simulink model "ClassDemo"  (R2014b)
settings: Solver=ode45  StartTime=0.0  StopTime=140  MaxStep=0.1  RelTol=1e-3
libraries: simulink x1
settings Model: Creator=jeff  LastModifiedBy=jeff

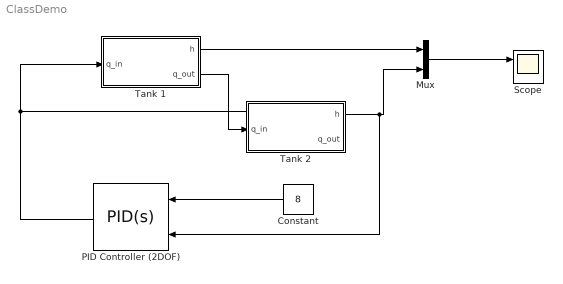
== system ClassDemo ==
  Constant : Constant  Value=8
  Mux : Mux  Inputs=2
  PID Controller (2DOF) : simulink/Continuous/PID Controller (2DOF)  Controller=PID  TimeDomain=Continuous-time  SampleTime=-1  IntegratorMethod=Forward Euler  FilterMethod=Forward Euler  Form=Parallel  P=0.2  I=0.01  D=2  N=100  b=1  c=0  InitialConditionSource=internal  InitialConditionForIntegrator=0  InitialConditionForFilter=0  ExternalReset=none  LimitOutput=off  UpperSaturationLimit=inf  LowerSaturationLimit=-inf  LinearizeAsGain=on  AntiWindupMode=none  Kb=1  TrackingMode=off  Kt=1  PParamMin=[]  PParamMax=[]  IParamMin=[]  IParamMax=[]  DParamMin=[]  DParamMax=[]  NParamMin=[]  NParamMax=[]  bParamMin=[]  bParamMax=[]  cParamMin=[]  cParamMax=[]  KbParamMin=[]  KbParamMax=[]  KtParamMin=[]  KtParamMax=[]  POutMin=[]  POutMax=[]  IOutMin=[]  IOutMax=[]  DOutMin=[]  DOutMax=[]  NOutMin=[]  NOutMax=[]  bOutMin=[]  bOutMax=[]  cOutMin=[]  cOutMax=[]  KbOutMin=[]  KbOutMax=[]  KtOutMin=[]  KtOutMax=[]  IntegratorOutMin=[]  IntegratorOutMax=[]  FilterOutMin=[]  FilterOutMax=[]  SumOutMin=[]  SumOutMax=[]  Sum1OutMin=[]  Sum1OutMax=[]  Sum2OutMin=[]  Sum2OutMax=[]  Sum3OutMin=[]  Sum3OutMax=[]  SumI1OutMin=[]  SumI1OutMax=[]  SumI2OutMin=[]  SumI2OutMax=[]  SumI3OutMin=[]  SumI3OutMax=[]  SumDOutMin=[]  SumDOutMax=[]  SaturationOutMin=[]  SaturationOutMax=[]  IntegratorContinuousStateAttributes=''  IntegratorStateMustResolveToSignalObject=off  IntegratorRTWStateStorageClass=Auto  FilterContinuousStateAttributes=''  FilterStateMustResolveToSignalObject=off  FilterRTWStateStorageClass=Auto  DifferentiatorICPrevScaledInput=0  DifferentiatorOutMin=[]  DifferentiatorOutMax=[]  UseFilter=on
  Scope : Scope  NumInputPorts=2
      settings: ShowLegends=on  TimeRange=167.6813022470671  YMin=0~-5  YMax=10~5
  Tank 1 : Subsystem
  Tank 2 : Subsystem
  wires:
  Tank 1/1(h) -> Mux/1
  Tank 1/2(q_out) -> Tank 2/1(q_in)
  Tank 2/1(h) -> PID Controller (2DOF)/2, Mux/2
  Mux/1 -> Scope/1
  Constant/1 -> PID Controller (2DOF)/1
  PID Controller (2DOF)/1 -> Tank 1/1(q_in)

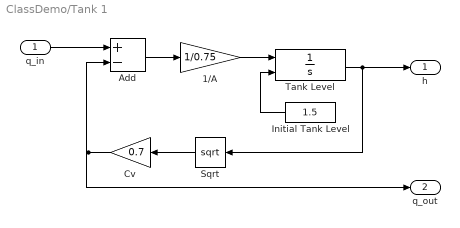
== system ClassDemo/Tank 1 ==
  q_in : Inport
  "1/A " : Gain  Gain=1/0.75
  Add : Sum  Inputs=+-
  Cv : Gain  Gain=0.7
  Initial Tank Level : Constant  Value=1.5
  Sqrt : Sqrt  SaturateOnIntegerOverflow=on
  Tank Level : Integrator  InitialConditionSource=external  LimitOutput=on  LowerSaturationLimit=0
  h : Outport
  q_out : Outport  Port=2
  wires:
  Tank Level/1 -> h/1, Sqrt/1
  Initial Tank Level/1 -> Tank Level/2
  "1/A "/1 -> Tank Level/1
  Cv/1 -> q_out/1, Add/2
  q_in/1 -> Add/1
  Add/1 -> "1/A "/1
  Sqrt/1 -> Cv/1

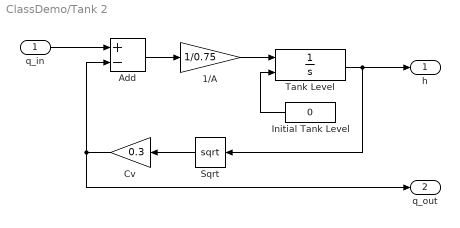
== system ClassDemo/Tank 2 ==
  q_in : Inport
  "1/A " : Gain  Gain=1/0.75
  Add : Sum  Inputs=+-
  Cv : Gain  Gain=0.3
  Initial Tank Level : Constant  Value=0
  Sqrt : Sqrt  SaturateOnIntegerOverflow=on
  Tank Level : Integrator  InitialConditionSource=external  LimitOutput=on  LowerSaturationLimit=0
  h : Outport
  q_out : Outport  Port=2
  wires:
  Tank Level/1 -> h/1, Sqrt/1
  Initial Tank Level/1 -> Tank Level/2
  "1/A "/1 -> Tank Level/1
  Cv/1 -> q_out/1, Add/2
  q_in/1 -> Add/1
  Add/1 -> "1/A "/1
  Sqrt/1 -> Cv/1
